simulink model "integrator_ext_IC_reset_test_tmp"  (Simulink 8.3)
settings: Solver=ode3  StartTime=0.0  StopTime=10.0  RelTol=1e-3
undefined symbols (not defined in the file): DiscIntNeverNeededParam
settings Model: Creator=arnaud  LastModifiedBy=hbourbou
settings DataIOCC: SaveFormat=Structure
settings OptimizationCC: ExpressionDepthLimit=2147483647
settings DebuggingCC: FcnCallInpInsideContextMsg=EnableAllAsWarning  FrameProcessingCompatibilityMsg=error

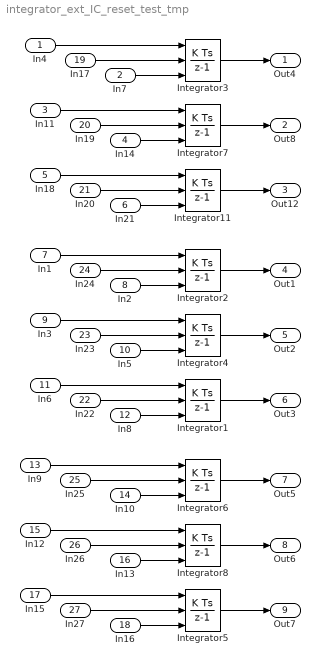
== system integrator_ext_IC_reset_test_tmp ==
  In4 : Inport  OutDataTypeStr=double
  In7 : Inport  Port=2  OutDataTypeStr=double
  In11 : Inport  Port=3  OutDataTypeStr=int32
  In14 : Inport  Port=4  OutDataTypeStr=int32
  In18 : Inport  Port=5  OutDataTypeStr=boolean
  In21 : Inport  Port=6  OutDataTypeStr=uint8
  In1 : Inport  Port=7  OutDataTypeStr=double
  In2 : Inport  Port=8  OutDataTypeStr=double
  In3 : Inport  Port=9  OutDataTypeStr=int32
  In5 : Inport  Port=10  OutDataTypeStr=int32
  In6 : Inport  Port=11  OutDataTypeStr=boolean
  In8 : Inport  Port=12  OutDataTypeStr=uint8
  In9 : Inport  Port=13  OutDataTypeStr=double
  In10 : Inport  Port=14  OutDataTypeStr=double
  In12 : Inport  Port=15  OutDataTypeStr=int32
  In13 : Inport  Port=16  OutDataTypeStr=int32
  In15 : Inport  Port=17  OutDataTypeStr=boolean
  In16 : Inport  Port=18  OutDataTypeStr=uint8
  In17 : Inport  Port=19  OutDataTypeStr=boolean
  In19 : Inport  Port=20  OutDataTypeStr=boolean
  In20 : Inport  Port=21  OutDataTypeStr=boolean
  In22 : Inport  Port=22  OutDataTypeStr=boolean
  In23 : Inport  Port=23  OutDataTypeStr=boolean
  In24 : Inport  Port=24  OutDataTypeStr=boolean
  In25 : Inport  Port=25  OutDataTypeStr=boolean
  In26 : Inport  Port=26  OutDataTypeStr=boolean
  In27 : Inport  Port=27  OutDataTypeStr=boolean
  Integrator1 : DiscreteIntegrator  ExternalReset=rising  InitialConditionSource=external  SampleTime=1.0  ICPrevOutput=DiscIntNeverNeededParam  ICPrevScaledInput=DiscIntNeverNeededParam  mask(DiscretizedDiscreteIntegrator){}
      mask init:
      | %zoh
  Integrator11 : DiscreteIntegrator  ExternalReset=rising  InitialConditionSource=external  SampleTime=1.0  ICPrevOutput=DiscIntNeverNeededParam  ICPrevScaledInput=DiscIntNeverNeededParam  mask(DiscretizedDiscreteIntegrator){}
      mask init:
      | %zoh
  Integrator2 : DiscreteIntegrator  ExternalReset=rising  InitialConditionSource=external  SampleTime=1.0  ICPrevOutput=DiscIntNeverNeededParam  ICPrevScaledInput=DiscIntNeverNeededParam  mask(DiscretizedDiscreteIntegrator){}
      mask init:
      | %zoh
  Integrator3 : DiscreteIntegrator  ExternalReset=rising  InitialConditionSource=external  SampleTime=1.0  ICPrevOutput=DiscIntNeverNeededParam  ICPrevScaledInput=DiscIntNeverNeededParam  mask(DiscretizedDiscreteIntegrator){}
      mask init:
      | %zoh
  Integrator4 : DiscreteIntegrator  ExternalReset=rising  InitialConditionSource=external  SampleTime=1.0  ICPrevOutput=DiscIntNeverNeededParam  ICPrevScaledInput=DiscIntNeverNeededParam  mask(DiscretizedDiscreteIntegrator){}
      mask init:
      | %zoh
  Integrator5 : DiscreteIntegrator  ExternalReset=rising  InitialConditionSource=external  SampleTime=1.0  ICPrevOutput=DiscIntNeverNeededParam  ICPrevScaledInput=DiscIntNeverNeededParam  mask(DiscretizedDiscreteIntegrator){}
      mask init:
      | %zoh
  Integrator6 : DiscreteIntegrator  ExternalReset=rising  InitialConditionSource=external  SampleTime=1.0  ICPrevOutput=DiscIntNeverNeededParam  ICPrevScaledInput=DiscIntNeverNeededParam  mask(DiscretizedDiscreteIntegrator){}
      mask init:
      | %zoh
  Integrator7 : DiscreteIntegrator  ExternalReset=rising  InitialConditionSource=external  SampleTime=1.0  ICPrevOutput=DiscIntNeverNeededParam  ICPrevScaledInput=DiscIntNeverNeededParam  mask(DiscretizedDiscreteIntegrator){}
      mask init:
      | %zoh
  Integrator8 : DiscreteIntegrator  ExternalReset=rising  InitialConditionSource=external  SampleTime=1.0  ICPrevOutput=DiscIntNeverNeededParam  ICPrevScaledInput=DiscIntNeverNeededParam  mask(DiscretizedDiscreteIntegrator){}
      mask init:
      | %zoh
  Out4 : Outport
  Out8 : Outport  Port=2
  Out12 : Outport  Port=3
  Out1 : Outport  Port=4
  Out2 : Outport  Port=5
  Out3 : Outport  Port=6
  Out5 : Outport  Port=7
  Out6 : Outport  Port=8
  Out7 : Outport  Port=9
  wires:
  In4/1 -> Integrator3/1
  Integrator3/1 -> Out4/1
  In7/1 -> Integrator3/3
  In11/1 -> Integrator7/1
  Integrator7/1 -> Out8/1
  In14/1 -> Integrator7/3
  In18/1 -> Integrator11/1
  Integrator11/1 -> Out12/1
  In21/1 -> Integrator11/3
  In1/1 -> Integrator2/1
  Integrator2/1 -> Out1/1
  In2/1 -> Integrator2/3
  In3/1 -> Integrator4/1
  Integrator4/1 -> Out2/1
  In5/1 -> Integrator4/3
  In6/1 -> Integrator1/1
  Integrator1/1 -> Out3/1
  In8/1 -> Integrator1/3
  In9/1 -> Integrator6/1
  Integrator6/1 -> Out5/1
  In10/1 -> Integrator6/3
  In12/1 -> Integrator8/1
  Integrator8/1 -> Out6/1
  In13/1 -> Integrator8/3
  In15/1 -> Integrator5/1
  Integrator5/1 -> Out7/1
  In16/1 -> Integrator5/3
  In17/1 -> Integrator3/2
  In19/1 -> Integrator7/2
  In20/1 -> Integrator11/2
  In22/1 -> Integrator1/2
  In23/1 -> Integrator4/2
  In24/1 -> Integrator2/2
  In25/1 -> Integrator6/2
  In26/1 -> Integrator8/2
  In27/1 -> Integrator5/2
